simulink model "ACDCMG_sim8"  (R2019b)
settings: Solver=ode8  StartTime=0.0  StopTime=0.5  FixedStep=40e-6  MaxStep=1e-2  RelTol=1e-3
InitFcn:
  | Set_parameters_R2018
undefined symbols (not defined in the file): D1, Delta, dis11, dis12, dis2, dis3, dis4, dis5, dis6, DiscIntNeverNeededParam, fn, Fnom, Ion, Lithium, max_min, P_Load_3, Pnom_T1, Pnom_T2, Pnom_T3, Ql_Load_3, R_Load_9, R_Load_DC, Rl, Rls, Ts, Ts_Control, Ts_Power, Ts_PV, V1_LL_T3, Vmin_mppt, VnInv, Vnom_DC, Vnom_Diesel, Vnom_prim, Vnom_sec, Vnom_ter_AC_DC, Xl, Xls
libraries: powerlib x133, powerlib_meascontrol x67, rtlab x23, simulink x7, powerlib_extras x5, electricdrivelib x1, eeSinusoidalMeasurementV2 x1, re_lib x1
(part 1 of 5)
settings Model: Creator=Leony  LastModifiedBy=dkh20
settings SolverCC: ZeroCrossAlgorithm=Adaptive  SolverResetMethod=Robust
settings DataIOCC: LimitDataPoints=on  SaveFormat=Array  ReturnWorkspaceOutputs=off
settings OptimizationCC: LifeSpan=inf
settings DebuggingCC: UnderspecifiedInitializationDetection=Classic  MergeDetectMultiDrivingBlocksExec=none  IgnoredZcDiagnostic=none  SolverPrmCheckMsg=warning  AllowSymbolicDim=off  SFUnexpectedBacktrackingDiag=warning  SFNoUnconditionalDefaultTransitionDiag=warning  SFExecutionAtInitializationDiag=none  ArithmeticOperatorsInVariantConditions=warning
settings HardwareCC: ProdBitPerPointer=32  ProdBitPerSizeT=32  ProdBitPerPtrDiffT=32  ProdLargestAtomicFloat=None  ProdIntDivRoundTo=Undefined  ProdEndianess=Unspecified  ProdWordSize=32  ProdHWDeviceType=32-bit Generic
settings ModelReferenceCC: PropagateSignalLabelsOutOfModel=off
settings SFSimCC: SimUseLocalCustomCode=off  CustomCodeUndefinedFunction=UseInterfaceOnly
settings RTWCC: RTWUseLocalCustomCode=off
settings CodeAppCC: StateflowObjectComments=on
settings GRTTargetCC: TargetLangStandard=C89/C90 (ANSI)
settings ConfigComp: CovMetricSettings=dw  CovSaveCumulativeToWorkspaceVar=on  CovSaveSingleToWorkspaceVar=on  CovExternalEMLEnable=off
settings SimscapeCC: SimscapeNormalizeSystem=off

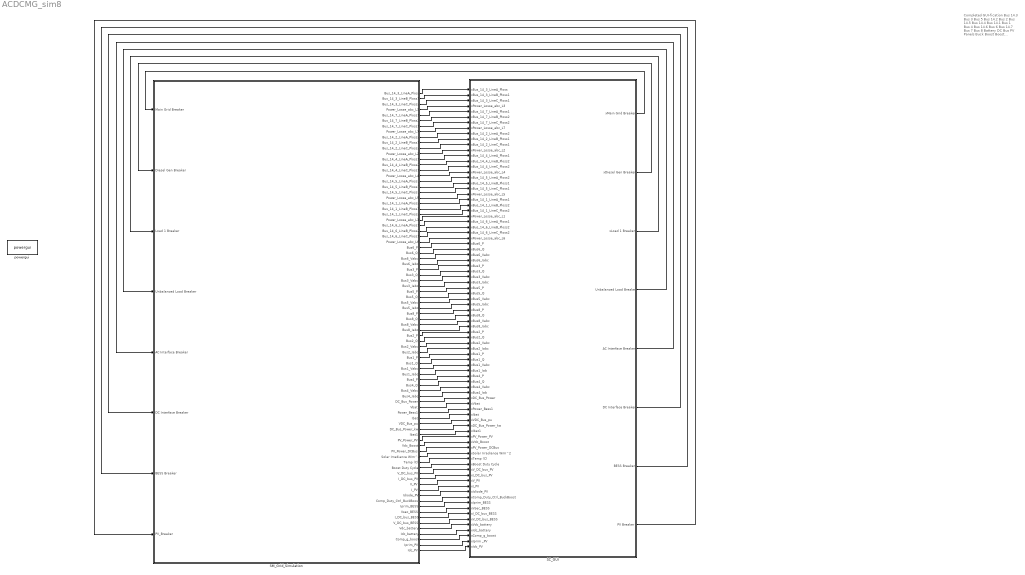
== system ACDCMG_sim8 ==
  note: Completed GUI-fication
      |
      | Bus 14.3
      | Bus 3
      | Bus 5
      | Bus 14.2
      | Bus 2
      | Bus 14.5
      | Bus 14.4
      | Bus 14.1
      | Bus 1
      | Bus 4
      | Bus 14.6
      | Bus 6
      | Bus 14.7
      | Bus 7
      | Bus 8
      | Battery
      | DC Bus
      | PV Panels
      | Buck Boost
      | Boost
      | Inverter
  SC_GUI : Subsystem
  SM_Grid_Simulation : Subsystem
  powergui : powerlib/powergui  Priority=1  SimulationMode=Discrete  SampleTime=Ts_Power  frequency=60  Iterations=50  frequencyindice=0  Pbase=100e6  ErrMax=1e-4  UnitsV=kV  UnitsW=MW  buscounter=0  FunctionMessages=off  echomessages=off  EnableUseOfTLC=off  CurrentSourceSwitches=off  DisableSnubberDevices=off  DisableRonSwitches=off  DisableVfSwitches=off  DisplayEquations=off  AutomaticDiscreteSolvers=off  SolverType=Tustin/Backward Euler (TBE)  Interpol=off  ExternalGateDelay=off  methode=off  Ts=100  x0status=blocks  SPID=on  SwTol=0  HookPort=off  NonlinearTolerance=1e-4  nMaxIteration=100  ContinueOnMaxIteration=off  RestoreLinks=warning  ResistiveCurrentMeasurement=off  Frange=[0:2:500]  Ylog=off  Xlog=on  ShowGrid=off  save=off  variable=ZData  structure=0  ZoomFFT=off  StartTime=0.0  cycles=1  DisplayStyle=1  fundamental=60  FreqAxis=off  MaxFrequency=1000  frequencyindicesteady=1  RmsSteady=1  display=off
      settings: SourceProductName=Simscape Electrical
  wires:
  SM_Grid_Simulation/1(Bus_14_3_LineA_Ploss) -> SC_GUI/1(xBus_14_3_LineA_Ploss)
  SM_Grid_Simulation/2(Bus_14_3_LineB_Ploss1) -> SC_GUI/2(xBus_14_3_LineB_Ploss1)
  SM_Grid_Simulation/3(Bus_14_3_LineC_Ploss2) -> SC_GUI/3(xBus_14_3_LineC_Ploss1)
  SM_Grid_Simulation/4(Power_Losse_abc_L3) -> SC_GUI/4(xPower_Losse_abc_L3)
  SM_Grid_Simulation/5(Bus_14_7_LineA_Ploss1) -> SC_GUI/5(xBus_14_7_LineA_Ploss1)
  SM_Grid_Simulation/6(Bus_14_7_LineB_Ploss2) -> SC_GUI/6(xBus_14_7_LineB_Ploss2)
  SM_Grid_Simulation/7(Bus_14_7_LineC_Ploss1) -> SC_GUI/7(xBus_14_7_LineC_Ploss2)
  SM_Grid_Simulation/8(Power_Losse_abc_L7) -> SC_GUI/8(xPower_Losse_abc_L7)
  SM_Grid_Simulation/9(Bus_14_2_LineA_Ploss2) -> SC_GUI/9(xBus_14_2_LineA_Ploss2)
  SM_Grid_Simulation/10(Bus_14_2_LineB_Ploss1) -> SC_GUI/10(xBus_14_2_LineB_Ploss1)
  SM_Grid_Simulation/11(Bus_14_2_LineC_Ploss2) -> SC_GUI/11(xBus_14_2_LineC_Ploss1)
  SM_Grid_Simulation/12(Power_Losse_abc_L2) -> SC_GUI/12(xPower_Losse_abc_L2)
  SM_Grid_Simulation/13(Bus_14_4_LineA_Ploss1) -> SC_GUI/13(xBus_14_4_LineA_Ploss1)
  SM_Grid_Simulation/14(Bus_14_4_LineB_Ploss2) -> SC_GUI/14(xBus_14_4_LineB_Ploss2)
  SM_Grid_Simulation/15(Bus_14_4_LineC_Ploss1) -> SC_GUI/15(xBus_14_4_LineC_Ploss2)
  SM_Grid_Simulation/16(Power_Losse_abc_L4) -> SC_GUI/16(xPower_Losse_abc_L4)
  SM_Grid_Simulation/17(Bus_14_5_LineA_Ploss3) -> SC_GUI/17(xBus_14_5_LineA_Ploss2)
  SM_Grid_Simulation/18(Bus_14_5_LineB_Ploss3) -> SC_GUI/18(xBus_14_5_LineB_Ploss1)
  SM_Grid_Simulation/19(Bus_14_5_LineC_Ploss3) -> SC_GUI/19(xBus_14_5_LineC_Ploss1)
  SM_Grid_Simulation/20(Power_Losse_abc_L5) -> SC_GUI/20(xPower_Losse_abc_L5)
  SM_Grid_Simulation/21(Bus_14_1_LineA_Ploss2) -> SC_GUI/21(xBus_14_1_LineA_Ploss1)
  SM_Grid_Simulation/22(Bus_14_1_LineB_Ploss1) -> SC_GUI/22(xBus_14_1_LineB_Ploss2)
  SM_Grid_Simulation/23(Bus_14_1_LineC_Ploss2) -> SC_GUI/23(xBus_14_1_LineC_Ploss2)
  SM_Grid_Simulation/24(Power_Losse_abc_L1) -> SC_GUI/24(xPower_Losse_abc_L1)
  SM_Grid_Simulation/25(Bus_14_6_LineA_Ploss1) -> SC_GUI/25(xBus_14_6_LineA_Ploss1)
  SM_Grid_Simulation/26(Bus_14_6_LineB_Ploss2) -> SC_GUI/26(xBus_14_6_LineB_Ploss2)
  SM_Grid_Simulation/27(Bus_14_6_LineC_Ploss1) -> SC_GUI/27(xBus_14_6_LineC_Ploss2)
  SM_Grid_Simulation/28(Power_Losse_abc_L6) -> SC_GUI/28(xPower_Losse_abc_L6)
  SM_Grid_Simulation/29(Bus6_P) -> SC_GUI/29(xBus6_P)
  SM_Grid_Simulation/30(Bus6_Q) -> SC_GUI/30(xBus6_Q)
  SM_Grid_Simulation/31(Bus6_Vabc) -> SC_GUI/31(xBus6_Vabc)
  SM_Grid_Simulation/32(Bus6_Iabc) -> SC_GUI/32(xBus6_Iabc)
  SM_Grid_Simulation/33(Bus3_P) -> SC_GUI/33(xBus3_P)
  SM_Grid_Simulation/34(Bus3_Q) -> SC_GUI/34(xBus3_Q)
  SM_Grid_Simulation/35(Bus3_Vabc) -> SC_GUI/35(xBus3_Vabc)
  SM_Grid_Simulation/36(Bus3_Iabc) -> SC_GUI/36(xBus3_Iabc)
  SM_Grid_Simulation/37(Bus5_P) -> SC_GUI/37(xBus5_P)
  SM_Grid_Simulation/38(Bus5_Q) -> SC_GUI/38(xBus5_Q)
  SM_Grid_Simulation/39(Bus5_Vabc) -> SC_GUI/39(xBus5_Vabc)
  SM_Grid_Simulation/40(Bus5_Iabc) -> SC_GUI/40(xBus5_Iabc)
  SM_Grid_Simulation/41(Bus8_P) -> SC_GUI/41(xBus8_P)
  SM_Grid_Simulation/42(Bus8_Q) -> SC_GUI/42(xBus8_Q)
  SM_Grid_Simulation/43(Bus8_Vabc) -> SC_GUI/43(xBus8_Vabc)
  SM_Grid_Simulation/44(Bus8_Iabc) -> SC_GUI/44(xBus8_Iabc)
  SM_Grid_Simulation/45(Bus2_P) -> SC_GUI/45(xBus2_P)
  SM_Grid_Simulation/46(Bus2_Q) -> SC_GUI/46(xBus2_Q)
  SM_Grid_Simulation/47(Bus2_Vabc) -> SC_GUI/47(xBus2_Vabc)
  SM_Grid_Simulation/48(Bus2_Iabc) -> SC_GUI/48(xBus2_Iabc)
  SM_Grid_Simulation/49(Bus1_P) -> SC_GUI/49(xBus1_P)
  SM_Grid_Simulation/50(Bus1_Q) -> SC_GUI/50(xBus1_Q)
  SM_Grid_Simulation/51(Bus1_Vabc) -> SC_GUI/51(xBus1_Vabc)
  SM_Grid_Simulation/52(Bus1_Iabc) -> SC_GUI/52(xBus1_Iab)
  SM_Grid_Simulation/53(Bus4_P) -> SC_GUI/53(xBus4_P)
  SM_Grid_Simulation/54(Bus4_Q) -> SC_GUI/54(xBus4_Q)
  SM_Grid_Simulation/55(Bus4_Vabc) -> SC_GUI/55(xBus4_Vabc)
  SM_Grid_Simulation/56(Bus4_Iabc) -> SC_GUI/56(xBus4_Iab)
  SM_Grid_Simulation/57(DC_Bus_Power) -> SC_GUI/57(xDC_Bus_Power)
  SM_Grid_Simulation/58(Vbat) -> SC_GUI/58(xVbat)
  SM_Grid_Simulation/59(Power_Bess1) -> SC_GUI/59(xPower_Bess1)
  SM_Grid_Simulation/60(Ibat) -> SC_GUI/60(xIbat)
  SM_Grid_Simulation/61(VDC_Bus_pu) -> SC_GUI/61(xVDC_Bus_pu)
  SM_Grid_Simulation/62(DC_Bus_Power_kw) -> SC_GUI/62(xDC_Bus_Power_kw)
  SM_Grid_Simulation/63(Ibat1) -> SC_GUI/63(xIbat1)
  SM_Grid_Simulation/64(PV_Power_PV) -> SC_GUI/64(xPV_Power_PV)
  SM_Grid_Simulation/65(Vdc_Boost) -> SC_GUI/65(xVdc_Boost)
  SM_Grid_Simulation/66(PV_Power_DCBus) -> SC_GUI/66(xPV_Power_DCBus)
  SM_Grid_Simulation/67(Solar Irradiance W/m^2) -> SC_GUI/67(xSolar Irradiance W/m^2)
  SM_Grid_Simulation/68(Temp (C)) -> SC_GUI/68(xTemp (C))
  SM_Grid_Simulation/69(Boost Duty Cycle) -> SC_GUI/69(xBoost Duty Cycle)
  SM_Grid_Simulation/70(V_DC_bus_PV) -> SC_GUI/70(xV_DC_bus_PV)
  SM_Grid_Simulation/71(I_DC_bus_PV) -> SC_GUI/71(xI_DC_bus_PV)
  SM_Grid_Simulation/72(V_PV) -> SC_GUI/72(xV_PV)
  SM_Grid_Simulation/73(I_PV) -> SC_GUI/73(xI_PV)
  SM_Grid_Simulation/74(Idiode_PV) -> SC_GUI/74(xIdiode_PV)
  SM_Grid_Simulation/75(Comp_Duty_Ctrl_BuckBoost) -> SC_GUI/75(xComp_Duty_Ctrl_BuckBoost)
  SM_Grid_Simulation/76(Iprim_BESS) -> SC_GUI/76(xIprim_BESS)
  SM_Grid_Simulation/77(Vsec_BESS) -> SC_GUI/77(xVsec_BESS)
  SM_Grid_Simulation/78(I_DC_bus_BESS) -> SC_GUI/78(xI_DC_bus_BESS)
  SM_Grid_Simulation/79(V_DC_bus_BESS) -> SC_GUI/79(xV_DC_bus_BESS)
  SM_Grid_Simulation/80(Vdc_battery) -> SC_GUI/80(xVdc_battery)
  SM_Grid_Simulation/81(Idc_battery) -> SC_GUI/81(xIdc_battery)
  SM_Grid_Simulation/82(Comp_g_boost) -> SC_GUI/82(xComp_g_boost)
  SM_Grid_Simulation/83(Iprim_PV) -> SC_GUI/83(xIprim _PV)
  SM_Grid_Simulation/84(Idc_PV) -> SC_GUI/84(xIdc_PV)
  SC_GUI/1(xMain Grid Breaker) -> SM_Grid_Simulation/1(Main Grid Breaker)
  SC_GUI/2(xDiesel Gen Breaker) -> SM_Grid_Simulation/2(Diesel Gen Breaker)
  SC_GUI/3(xLoad 1 Breaker) -> SM_Grid_Simulation/3(Load 1 Breaker)
  SC_GUI/4(Unbalanced Load Breaker) -> SM_Grid_Simulation/4(Unbalanced Load Breaker)
  SC_GUI/5(AC Interface Breaker) -> SM_Grid_Simulation/5(AC Interface Breaker)
  SC_GUI/6(DC Interface Breaker) -> SM_Grid_Simulation/6(DC Interface Breaker)
  SC_GUI/7(BESS Breaker) -> SM_Grid_Simulation/7(BESS Breaker)
  SC_GUI/8(PV Breaker) -> SM_Grid_Simulation/8(PV_Breaker)

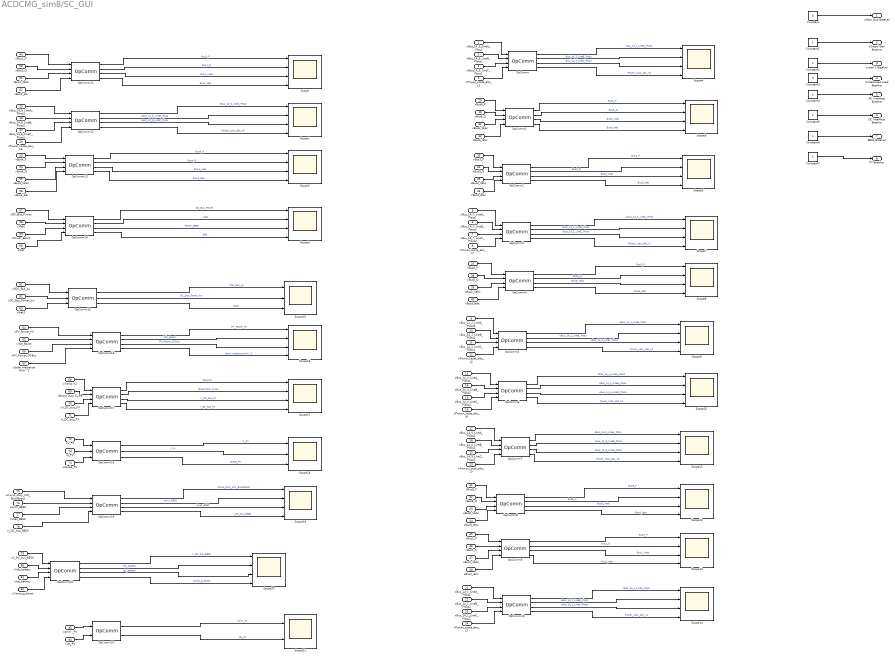
== system ACDCMG_sim8/SC_GUI ==
  xBus_14_3_LineA_Ploss : Inport
  xBus_14_3_LineB_Ploss1 : Inport  Port=2
  xBus_14_3_LineC_Ploss1 : Inport  Port=3
  xPower_Losse_abc_L3 : Inport  Port=4
  xBus_14_7_LineA_Ploss1 : Inport  Port=5
  xBus_14_7_LineB_Ploss2 : Inport  Port=6
  xBus_14_7_LineC_Ploss2 : Inport  Port=7
  xPower_Losse_abc_L7 : Inport  Port=8
  xBus_14_2_LineA_Ploss2 : Inport  Port=9
  xBus_14_2_LineB_Ploss1 : Inport  Port=10
  xBus_14_2_LineC_Ploss1 : Inport  Port=11
  xPower_Losse_abc_L2 : Inport  Port=12
  xBus_14_4_LineA_Ploss1 : Inport  Port=13
  xBus_14_4_LineB_Ploss2 : Inport  Port=14
  xBus_14_4_LineC_Ploss2 : Inport  Port=15
  xPower_Losse_abc_L4 : Inport  Port=16
  xBus_14_5_LineA_Ploss2 : Inport  Port=17
  xBus_14_5_LineB_Ploss1 : Inport  Port=18
  xBus_14_5_LineC_Ploss1 : Inport  Port=19
  xPower_Losse_abc_L5 : Inport  Port=20
  xBus_14_1_LineA_Ploss1 : Inport  Port=21
  xBus_14_1_LineB_Ploss2 : Inport  Port=22
  xBus_14_1_LineC_Ploss2 : Inport  Port=23
  xPower_Losse_abc_L1 : Inport  Port=24
  xBus_14_6_LineA_Ploss1 : Inport  Port=25
  xBus_14_6_LineB_Ploss2 : Inport  Port=26
  xBus_14_6_LineC_Ploss2 : Inport  Port=27
  xPower_Losse_abc_L6 : Inport  Port=28
  xBus6_P : Inport  Port=29
  xBus6_Q : Inport  Port=30
  xBus6_Vabc : Inport  Port=31
  xBus6_Iabc : Inport  Port=32
  xBus3_P : Inport  Port=33
  xBus3_Q : Inport  Port=34
  xBus3_Vabc : Inport  Port=35
  xBus3_Iabc : Inport  Port=36
  xBus5_P : Inport  Port=37
  xBus5_Q : Inport  Port=38
  xBus5_Vabc : Inport  Port=39
  xBus5_Iabc : Inport  Port=40
  xBus8_P : Inport  Port=41
  xBus8_Q : Inport  Port=42
  xBus8_Vabc : Inport  Port=43
  xBus8_Iabc : Inport  Port=44
  xBus2_P : Inport  Port=45
  xBus2_Q : Inport  Port=46
  xBus2_Vabc : Inport  Port=47
  xBus2_Iabc : Inport  Port=48
  xBus1_P : Inport  Port=49
  xBus1_Q : Inport  Port=50
  xBus1_Vabc : Inport  Port=51
  xBus1_Iab : Inport  Port=52
  xBus4_P : Inport  Port=53
  xBus4_Q : Inport  Port=54
  xBus4_Vabc : Inport  Port=55
  xBus4_Iab : Inport  Port=56
  xDC_Bus_Power : Inport  Port=57
  xVbat : Inport  Port=58
  xPower_Bess1 : Inport  Port=59
  xIbat : Inport  Port=60
  xVDC_Bus_pu : Inport  Port=61
  xDC_Bus_Power_kw : Inport  Port=62
  xIbat1 : Inport  Port=63
  xPV_Power_PV : Inport  Port=64
  xVdc_Boost : Inport  Port=65
  xPV_Power_DCBus : Inport  Port=66
  xSolar Irradiance W/m^2 : Inport  Port=67
  xTemp (C) : Inport  Port=68
  xBoost Duty Cycle : Inport  Port=69
  xV_DC_bus_PV : Inport  Port=70
  xI_DC_bus_PV : Inport  Port=71
  xV_PV : Inport  Port=72
  xI_PV : Inport  Port=73
  xIdiode_PV : Inport  Port=74
  xComp_Duty_Ctrl_BuckBoost : Inport  Port=75
  xIprim_BESS : Inport  Port=76
  xVsec_BESS : Inport  Port=77
  xI_DC_bus_BESS : Inport  Port=78
  xV_DC_bus_BESS : Inport  Port=79
  xVdc_battery : Inport  Port=80
  xIdc_battery : Inport  Port=81
  xComp_g_boost : Inport  Port=82
  xIprim _PV : Inport  Port=83
  xIdc_PV : Inport  Port=84
  Constant : Constant  Value=0
  Constant{1..2,4..7} (6 alike) : Constant
  Constant3 : Constant  Value=0
  OpComm : rtlab/OpComm  nbport=4  groupe_acq=1  subsys_rate=0  st=0  Synchronization=on  Interpolation=on  Threshold=1.0  Missed_Data=off  Sim_Time=off  Samples=off  dynSigOut=off  from_console=0  warning_done=off  writeOpCommFile=off  Offset=off
      settings: SourceProductName=RT-LAB
  OpComm1 : rtlab/OpComm  nbport=4  groupe_acq=2  subsys_rate=0  st=0  Synchronization=on  Interpolation=on  Threshold=1.0  Missed_Data=off  Sim_Time=off  Samples=off  dynSigOut=off  from_console=0  warning_done=off  writeOpCommFile=off  Offset=off
      settings: SourceProductName=RT-LAB
  OpComm10 : rtlab/OpComm  nbport=4  groupe_acq=11  subsys_rate=0  st=0  Synchronization=on  Interpolation=on  Threshold=1.0  Missed_Data=off  Sim_Time=off  Samples=off  dynSigOut=off  from_console=0  warning_done=off  writeOpCommFile=off  Offset=off
      settings: SourceProductName=RT-LAB
  OpComm11 : rtlab/OpComm  nbport=4  groupe_acq=12  subsys_rate=0  st=0  Synchronization=on  Interpolation=on  Threshold=1.0  Missed_Data=off  Sim_Time=off  Samples=off  dynSigOut=off  from_console=0  warning_done=off  writeOpCommFile=off  Offset=off
      settings: SourceProductName=RT-LAB
  OpComm12 : rtlab/OpComm  nbport=4  groupe_acq=13  subsys_rate=0  st=0  Synchronization=on  Interpolation=on  Threshold=1.0  Missed_Data=off  Sim_Time=off  Samples=off  dynSigOut=off  from_console=0  warning_done=off  writeOpCommFile=off  Offset=off
      settings: SourceProductName=RT-LAB
  OpComm13 : rtlab/OpComm  nbport=4  groupe_acq=14  subsys_rate=0  st=0  Synchronization=on  Interpolation=on  Threshold=1.0  Missed_Data=off  Sim_Time=off  Samples=off  dynSigOut=off  from_console=0  warning_done=off  writeOpCommFile=off  Offset=off
      settings: SourceProductName=RT-LAB
  OpComm14 : rtlab/OpComm  nbport=4  groupe_acq=16  subsys_rate=0  st=0  Synchronization=on  Interpolation=on  Threshold=1.0  Missed_Data=off  Sim_Time=off  Samples=off  dynSigOut=off  from_console=0  warning_done=off  writeOpCommFile=off  Offset=off
      settings: SourceProductName=RT-LAB
  OpComm15 : rtlab/OpComm  nbport=3  groupe_acq=17  subsys_rate=0  st=0  Synchronization=on  Interpolation=on  Threshold=1.0  Missed_Data=off  Sim_Time=off  Samples=off  dynSigOut=off  from_console=0  warning_done=off  writeOpCommFile=off  Offset=off
      settings: SourceProductName=RT-LAB
  OpComm16 : rtlab/OpComm  nbport=4  groupe_acq=18  subsys_rate=0  st=0  Synchronization=on  Interpolation=on  Threshold=1.0  Missed_Data=off  Sim_Time=off  Samples=off  dynSigOut=off  from_console=0  warning_done=off  writeOpCommFile=off  Offset=off
      settings: SourceProductName=RT-LAB
  OpComm17 : rtlab/OpComm  nbport=4  groupe_acq=19  subsys_rate=0  st=0  Synchronization=on  Interpolation=on  Threshold=1.0  Missed_Data=off  Sim_Time=off  Samples=off  dynSigOut=off  from_console=0  warning_done=off  writeOpCommFile=off  Offset=off
      settings: SourceProductName=RT-LAB
  OpComm18 : rtlab/OpComm  nbport=3  groupe_acq=20  subsys_rate=0  st=0  Synchronization=on  Interpolation=on  Threshold=1.0  Missed_Data=off  Sim_Time=off  Samples=off  dynSigOut=off  from_console=0  warning_done=off  writeOpCommFile=off  Offset=off
      settings: SourceProductName=RT-LAB
  OpComm19 : rtlab/OpComm  nbport=4  groupe_acq=21  subsys_rate=0  st=0  Synchronization=on  Interpolation=on  Threshold=1.0  Missed_Data=off  Sim_Time=off  Samples=off  dynSigOut=off  from_console=0  warning_done=off  writeOpCommFile=off  Offset=off
      settings: SourceProductName=RT-LAB
  OpComm2 : rtlab/OpComm  nbport=4  groupe_acq=3  subsys_rate=0  st=0  Synchronization=on  Interpolation=on  Threshold=1.0  Missed_Data=off  Sim_Time=off  Samples=off  dynSigOut=off  from_console=0  warning_done=off  writeOpCommFile=off  Offset=off
      settings: SourceProductName=RT-LAB
  OpComm20 : rtlab/OpComm  nbport=4  groupe_acq=22  subsys_rate=0  st=0  Synchronization=on  Interpolation=on  Threshold=1.0  Missed_Data=off  Sim_Time=off  Samples=off  dynSigOut=off  from_console=0  warning_done=off  writeOpCommFile=off  Offset=off
      settings: SourceProductName=RT-LAB
  OpComm21 : rtlab/OpComm  nbport=2  groupe_acq=23  subsys_rate=0  st=0  Synchronization=on  Interpolation=on  Threshold=1.0  Missed_Data=off  Sim_Time=off  Samples=off  dynSigOut=off  from_console=0  warning_done=off  writeOpCommFile=off  Offset=off
      settings: SourceProductName=RT-LAB
  OpComm3 : rtlab/OpComm  nbport=4  groupe_acq=4  subsys_rate=0  st=0  Synchronization=on  Interpolation=on  Threshold=1.0  Missed_Data=off  Sim_Time=off  Samples=off  dynSigOut=off  from_console=0  warning_done=off  writeOpCommFile=off  Offset=off
      settings: SourceProductName=RT-LAB
  OpComm4 : rtlab/OpComm  nbport=4  groupe_acq=5  subsys_rate=0  st=0  Synchronization=on  Interpolation=on  Threshold=1.0  Missed_Data=off  Sim_Time=off  Samples=off  dynSigOut=off  from_console=0  warning_done=off  writeOpCommFile=off  Offset=off
      settings: SourceProductName=RT-LAB
  OpComm5 : rtlab/OpComm  nbport=4  groupe_acq=6  subsys_rate=0  st=0  Synchronization=on  Interpolation=on  Threshold=1.0  Missed_Data=off  Sim_Time=off  Samples=off  dynSigOut=off  from_console=0  warning_done=off  writeOpCommFile=off  Offset=off
      settings: SourceProductName=RT-LAB
  OpComm6 : rtlab/OpComm  nbport=4  groupe_acq=7  subsys_rate=0  st=0  Synchronization=on  Interpolation=on  Threshold=1.0  Missed_Data=off  Sim_Time=off  Samples=off  dynSigOut=off  from_console=0  warning_done=off  writeOpCommFile=off  Offset=off
      settings: SourceProductName=RT-LAB
  OpComm7 : rtlab/OpComm  nbport=4  groupe_acq=8  subsys_rate=0  st=0  Synchronization=on  Interpolation=on  Threshold=1.0  Missed_Data=off  Sim_Time=off  Samples=off  dynSigOut=off  from_console=0  warning_done=off  writeOpCommFile=off  Offset=off
      settings: SourceProductName=RT-LAB
  OpComm8 : rtlab/OpComm  nbport=4  groupe_acq=9  subsys_rate=0  st=0  Synchronization=on  Interpolation=on  Threshold=1.0  Missed_Data=off  Sim_Time=off  Samples=off  dynSigOut=off  from_console=0  warning_done=off  writeOpCommFile=off  Offset=off
      settings: SourceProductName=RT-LAB
  OpComm9 : rtlab/OpComm  nbport=4  groupe_acq=10  subsys_rate=0  st=0  Synchronization=on  Interpolation=on  Threshold=1.0  Missed_Data=off  Sim_Time=off  Samples=off  dynSigOut=off  from_console=0  warning_done=off  writeOpCommFile=off  Offset=off
      settings: SourceProductName=RT-LAB
  Scope{,1..14,16..17,19..20} (19 alike) : Scope  NumInputPorts=4
  Scope15 : Scope  NumInputPorts=3
  Scope18 : Scope  NumInputPorts=3
  Scope21 : Scope  NumInputPorts=2
  xMain Grid Breaker : Outport
  xDiesel Gen Breaker : Outport  Port=2
  xLoad 1 Breaker : Outport  Port=3
  Unbalanced Load Breaker : Outport  Port=4
  AC Interface Breaker : Outport  Port=5
  DC Interface Breaker : Outport  Port=6
  BESS Breaker : Outport  Port=7
  PV Breaker : Outport  Port=8
  wires:
  Constant/1 -> xMain Grid Breaker/1
  Constant1/1 -> xDiesel Gen Breaker/1
  Constant2/1 -> xLoad 1 Breaker/1
  Constant3/1 -> Unbalanced Load Breaker/1
  Constant4/1 -> AC Interface Breaker/1
  Constant5/1 -> DC Interface Breaker/1
  Constant6/1 -> BESS Breaker/1
  Constant7/1 -> PV Breaker/1
  xBus_14_3_LineA_Ploss/1 -> OpComm/1
  xBus_14_3_LineB_Ploss1/1 -> OpComm/2
  xBus_14_3_LineC_Ploss1/1 -> OpComm/3
  xPower_Losse_abc_L3/1 -> OpComm/4
  OpComm/1 -> Scope4/1  "Bus_14_3_LineA_Ploss"
  OpComm/2 -> Scope4/2  "Bus_14_3_LineB_Ploss"
  OpComm/3 -> Scope4/3  "Bus_14_3_LineC_Ploss"
  OpComm/4 -> Scope4/4  "Power_Loss_abc_L3"
  OpComm1/2 -> Scope5/2  "Bus6_Q"
  OpComm1/3 -> Scope5/3  "Bus6_Vabc"
  OpComm1/1 -> Scope5/1  "Bus6_P"
  OpComm1/4 -> Scope5/4  "Bus6_Iabc"
  xBus6_P/1 -> OpComm1/1
  xBus6_Q/1 -> OpComm1/2
  xBus6_Vabc/1 -> OpComm1/3
  xBus6_Iabc/1 -> OpComm1/4
  OpComm2/1 -> Scope6/1  "Bus3_P"
  OpComm2/2 -> Scope6/2  "Bus3_Q"
  OpComm2/3 -> Scope6/3  "Bus3_Vabc"
  OpComm2/4 -> Scope6/4  "Bus3_Iabc"
  xBus3_P/1 -> OpComm2/1
  xBus3_Q/1 -> OpComm2/2
  xBus3_Vabc/1 -> OpComm2/3
  xBus3_Iabc/1 -> OpComm2/4
  OpComm3/2 -> Scope7/2  "xBus_14_1_LineB_Ploss"
  OpComm3/3 -> Scope7/3  "xBus_14_1_LineC_Ploss"
  OpComm3/1 -> Scope7/1  "xBus_14_1_LineA_Ploss"
  OpComm3/4 -> Scope7/4  "Power_Loss_abc_L7"
  xBus_14_7_LineA_Ploss1/1 -> OpComm3/1
  xBus_14_7_LineB_Ploss2/1 -> OpComm3/2
  xBus_14_7_LineC_Ploss2/1 -> OpComm3/3
  xPower_Losse_abc_L7/1 -> OpComm3/4
  OpComm4/2 -> Scope8/2  "Bus5_Q"
  OpComm4/3 -> Scope8/3  "Bus5_Vabc"
  OpComm4/4 -> Scope8/4  "Bus5_Iabc"
  OpComm4/1 -> Scope8/1  "Bus5_P"
  xBus5_P/1 -> OpComm4/1
  xBus5_Q/1 -> OpComm4/2
  xBus5_Vabc/1 -> OpComm4/3
  xBus5_Iabc/1 -> OpComm4/4
  xBus_14_2_LineA_Ploss2/1 -> OpComm5/1
  xBus_14_2_LineB_Ploss1/1 -> OpComm5/2
  xBus_14_2_LineC_Ploss1/1 -> OpComm5/3
  xPower_Losse_abc_L2/1 -> OpComm5/4
  OpComm5/1 -> Scope9/1  "xBus_14_2_LineA_Ploss"
  OpComm5/2 -> Scope9/2  "xBus_14_2_LineB_Ploss"
  OpComm5/3 -> Scope9/3  "xBus_14_2_LineC_Ploss"
  OpComm5/4 -> Scope9/4  "Power_Loss_abc_L2"
  OpComm6/1 -> Scope10/1  "xBus_14_4_LineA_Ploss"
  OpComm6/2 -> Scope10/2  "xBus_14_4_LineB_Ploss"
  OpComm6/3 -> Scope10/3  "xBus_14_4_LineC_Ploss"
  OpComm6/4 -> Scope10/4  "Power_Loss_abc_L4"
  xBus_14_4_LineA_Ploss1/1 -> OpComm6/1
  xBus_14_4_LineB_Ploss2/1 -> OpComm6/2
  xBus_14_4_LineC_Ploss2/1 -> OpComm6/3
  xPower_Losse_abc_L4/1 -> OpComm6/4
  OpComm7/1 -> Scope11/1  "xBus_14_5_LineA_Ploss"
  OpComm7/2 -> Scope11/2  "xBus_14_5_LineB_Ploss"
  OpComm7/3 -> Scope11/3  "xBus_14_5_LineC_Ploss"
  OpComm7/4 -> Scope11/4  "Power_Loss_abc_L5"
  xBus_14_5_LineA_Ploss2/1 -> OpComm7/1
  xBus_14_5_LineB_Ploss1/1 -> OpComm7/2
  xBus_14_5_LineC_Ploss1/1 -> OpComm7/3
  xPower_Losse_abc_L5/1 -> OpComm7/4
  xBus8_P/1 -> OpComm8/1
  xBus8_Q/1 -> OpComm8/2
  xBus8_Vabc/1 -> OpComm8/3
  xBus8_Iabc/1 -> OpComm8/4
  OpComm8/1 -> Scope12/1  "Bus8_P"
  OpComm8/2 -> Scope12/2  "Bus8_Q"
  OpComm8/3 -> Scope12/3  "Bus8_Vabc"
  OpComm8/4 -> Scope12/4  "Bus8_Iabc"
  OpComm10/1 -> Scope14/1  "xBus_14_1_LineA_Ploss"
  OpComm10/2 -> Scope14/2  "xBus_14_1_LineB_Ploss"
  OpComm10/3 -> Scope14/3  "xBus_14_1_LineC_Ploss"
  OpComm10/4 -> Scope14/4  "Power_Loss_abc_L1"
  OpComm9/1 -> Scope13/1  "Bus2_P"
  OpComm9/2 -> Scope13/2  "Bus2_Q"
  OpComm9/3 -> Scope13/3  "Bus2_Vabc"
  OpComm9/4 -> Scope13/4  "Bus2_Iabc"
  xBus2_P/1 -> OpComm9/1
  xBus2_Q/1 -> OpComm9/2
  xBus2_Vabc/1 -> OpComm9/3
  xBus2_Iabc/1 -> OpComm9/4
  xBus_14_1_LineA_Ploss1/1 -> OpComm10/1
  xBus_14_1_LineB_Ploss2/1 -> OpComm10/2
  xBus_14_1_LineC_Ploss2/1 -> OpComm10/3
  xPower_Losse_abc_L1/1 -> OpComm10/4
  OpComm11/1 -> Scope/1  "Bus1_P"
  OpComm11/2 -> Scope/2  "Bus1_Q"
  OpComm11/3 -> Scope/3  "Bus1_Vabc"
  OpComm11/4 -> Scope/4  "Bus1_Iabc"
  xBus1_P/1 -> OpComm11/1
  xBus1_Q/1 -> OpComm11/2
  xBus1_Vabc/1 -> OpComm11/3
  xBus1_Iab/1 -> OpComm11/4
  OpComm12/1 -> Scope1/1  "xBus_14_6_LineA_Ploss"
  OpComm12/2 -> Scope1/2  "xBus_14_6_LineB_Ploss"
  OpComm12/3 -> Scope1/3  "xBus_14_6_LineC_Ploss"
  OpComm12/4 -> Scope1/4  "Power_Loss_abc_L6"
  xBus_14_6_LineA_Ploss1/1 -> OpComm12/1
  xBus_14_6_LineB_Ploss2/1 -> OpComm12/2
  xBus_14_6_LineC_Ploss2/1 -> OpComm12/3
  xPower_Losse_abc_L6/1 -> OpComm12/4
  xBus4_P/1 -> OpComm13/1
  xBus4_Q/1 -> OpComm13/2
  xBus4_Vabc/1 -> OpComm13/3
  xBus4_Iab/1 -> OpComm13/4
  OpComm13/1 -> Scope2/1  "Bus4_P"
  OpComm13/2 -> Scope2/2  "Bus4_Q"
  OpComm13/3 -> Scope2/3  "Bus4_Vabc"
  OpComm13/4 -> Scope2/4  "Bus4_Iabc"
  xDC_Bus_Power/1 -> OpComm14/1
  xVbat/1 -> OpComm14/2
  xPower_Bess1/1 -> OpComm14/3
  xIbat/1 -> OpComm14/4
  OpComm14/1 -> Scope3/1  "DC_Bus_Power"
  OpComm14/2 -> Scope3/2  "Vbat"
  OpComm14/3 -> Scope3/3  "Power_BESS"
  OpComm14/4 -> Scope3/4  "Ibat"
  xVDC_Bus_pu/1 -> OpComm15/1
  xDC_Bus_Power_kw/1 -> OpComm15/2
  xIbat1/1 -> OpComm15/3
  OpComm15/1 -> Scope15/1  "VDC_Bus_pu"
  OpComm15/2 -> Scope15/2  "DC_Bus_Power_kw"
  OpComm15/3 -> Scope15/3  "Ibat1"
  OpComm16/1 -> Scope16/1  "PV_Power_PV"
  OpComm16/2 -> Scope16/2  "Vdc_Boost"
  OpComm16/3 -> Scope16/3  "PV_Power_DCBus"
  OpComm16/4 -> Scope16/4  "Solar Irradiance W/m^2"
  xPV_Power_PV/1 -> OpComm16/1
  xVdc_Boost/1 -> OpComm16/2
  xPV_Power_DCBus/1 -> OpComm16/3
  xSolar Irradiance W/m^2/1 -> OpComm16/4
  OpComm17/1 -> Scope17/1  "Temp(C)"
  OpComm17/2 -> Scope17/2  "Boost Duty Cycle"
  OpComm17/3 -> Scope17/3  "V_DC_bus_PV"
  OpComm17/4 -> Scope17/4  "I_DC_bus_PV"
  xTemp (C)/1 -> OpComm17/1
  xBoost Duty Cycle/1 -> OpComm17/2
  xV_DC_bus_PV/1 -> OpComm17/3
  xI_DC_bus_PV/1 -> OpComm17/4
  OpComm18/1 -> Scope18/1  "V_PV"
  OpComm18/2 -> Scope18/2  "I_PV"
  OpComm18/3 -> Scope18/3  "Idiode_PV"
  xV_PV/1 -> OpComm18/1
  xI_PV/1 -> OpComm18/2
  xIdiode_PV/1 -> OpComm18/3
  OpComm19/1 -> Scope19/1  "Comp_Duty_Ctrl_BuckBoost"
  OpComm19/2 -> Scope19/2  "Iprim_BESS"
  OpComm19/3 -> Scope19/3  "Vsec_BESS"
  OpComm19/4 -> Scope19/4  "I_DC_bus_BESS"
  xComp_Duty_Ctrl_BuckBoost/1 -> OpComm19/1
  xIprim_BESS/1 -> OpComm19/2
  xVsec_BESS/1 -> OpComm19/3
  xI_DC_bus_BESS/1 -> OpComm19/4
  OpComm20/1 -> Scope20/1  "V_DC_bus_BESS"
  OpComm20/2 -> Scope20/2  "Vdc_battery"
  OpComm20/3 -> Scope20/3  "Idc_battery"
  OpComm20/4 -> Scope20/4  "Comp_g_boost"
  xV_DC_bus_BESS/1 -> OpComm20/1
  xVdc_battery/1 -> OpComm20/2
  xIdc_battery/1 -> OpComm20/3
  xComp_g_boost/1 -> OpComm20/4
  xIprim _PV/1 -> OpComm21/1
  OpComm21/1 -> Scope21/1  "Iprim_PV"
  OpComm21/2 -> Scope21/2  "Idc_PV"
  xIdc_PV/1 -> OpComm21/2
